simulink model "Speed_Control_Scalar"  (R2023b)
settings: Solver=ode3  StartTime=0.0  StopTime=20  FixedStep=1e-5  RelTol=1e-3
libraries: spsIGBTDiodeLib x6, spsCurrentMeasurementLib x3, spsAsynchronousMachineSIUnitsLib x1, spsDCVoltageSourceLib x1, slpidlib x1, simulink x1, spspowerguiLib x1
settings Model: Creator=G Nithish Chandra  LastModifiedBy=G Nithish Chandra

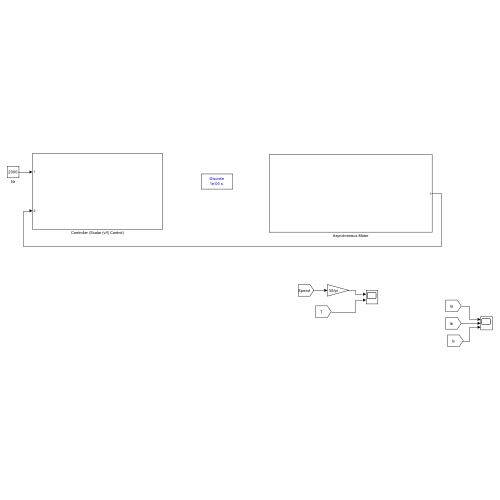
[thumbnail: Simulink's stored preview of the top-level diagram]
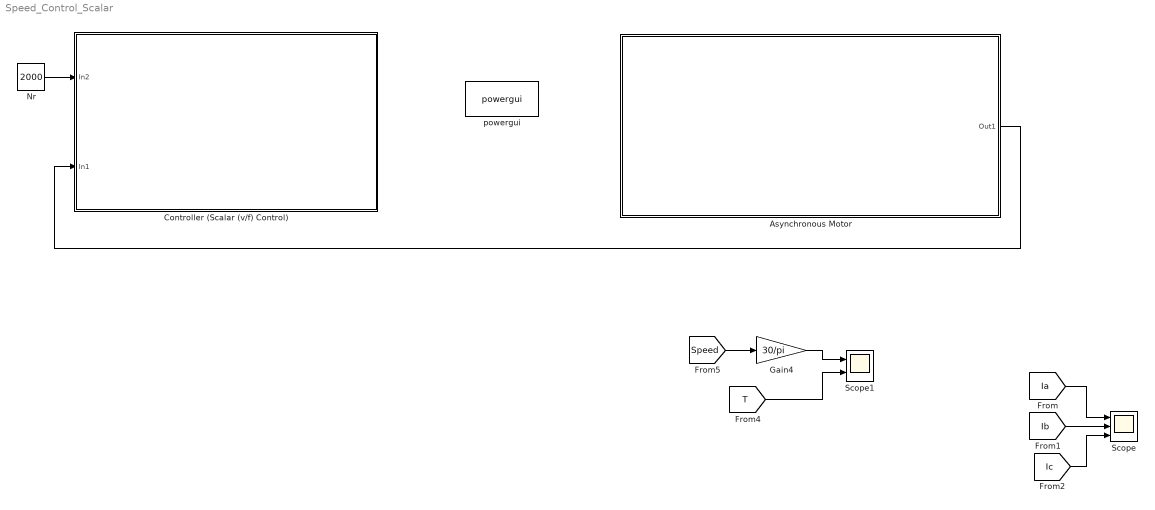
== system Speed_Control_Scalar ==
  Asynchronous Motor : Subsystem
  Controller (Scalar (v/f) Control) : Subsystem
  Gain4 : Gain  Gain=30/pi
  Nr : Constant  Value=2000
  Scope : Scope  NumInputPorts=3
  Scope1 : Scope  NumInputPorts=2
  powergui : spspowerguiLib/powergui  Priority=1  SimulationMode=Discrete  SampleTime=1e-5  frequency=60  Iterations=50  frequencyindice=50  Pbase=100e6  ErrMax=1e-4  UnitsV=kV  UnitsW=MW  buscounter=0  FunctionMessages=off  echomessages=off  EnableUseOfTLC=off  CurrentSourceSwitches=off  DisableSnubberDevices=off  DisableRonSwitches=off  DisableVfSwitches=off  DisplayEquations=off  AutomaticDiscreteSolvers=off  SolverType=Tustin/Backward Euler (TBE)  Interpol=off  ExternalGateDelay=off  methode=off  Ts=100  x0status=blocks  SPID=on  SwTol=0  HookPort=off  NonlinearTolerance=1e-4  nMaxIteration=100  ContinueOnMaxIteration=off  RestoreLinks=warning  ResistiveCurrentMeasurement=off  Frange=[0:2:500]  Ylog=off  Xlog=on  ShowGrid=off  save=off  variable=ZData  structure=0  ZoomFFT=off  StartTime=0.0  cycles=1  DisplayStyle=1  fundamental=60  FreqAxis=off  MaxFrequency=1000  frequencyindicesteady=1  RmsSteady=1  display=off
  wires:
  [Ia] -> Scope/1
  [Ic] -> Scope/3
  [Ib] -> Scope/2
  Asynchronous Motor/1(Out1) -> Controller (Scalar (v/f) Control)/2(In1)
  Nr/1 -> Controller (Scalar (v/f) Control)/1(In2)
  [Speed] -> Gain4/1
  Gain4/1 -> Scope1/1
  [T] -> Scope1/2

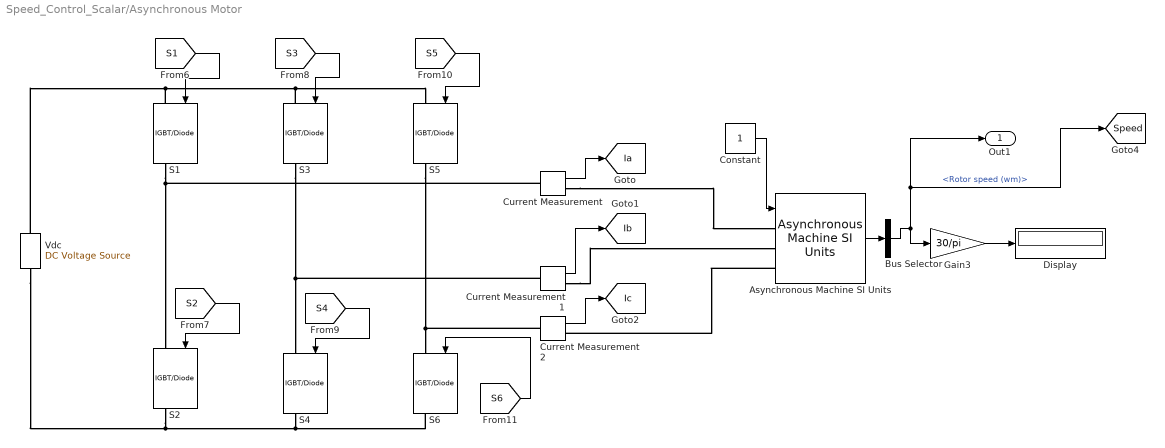
== system Speed_Control_Scalar/Asynchronous Motor ==
  Asynchronous Machine SI Units : spsAsynchronousMachineSIUnitsLib/Asynchronous Machine SI Units  RotorType=Squirrel-cage  PresetModel=No  MechanicalLoad=Torque Tm  ShowDetailedParameters=on  ReferenceFrame=Rotor  Units=SI  MeasurementBus=off  NominalParameters=[1.845e+04 400 50]  VoltageRatio=1  Stator=[0.5968 0.0003495]  Rotor=[0.6258 0.005473]  Cage1=[0.4155 0.002066]  Cage2=[0.4168 0.0003495]  Lm=0.0354  Mechanical=[0.05 0.005879 2]  PolePairs=2  InitialConditions=[0 0 0 0 0 0 0 0]  SimulateSaturation=off  Saturation=[14.03593122, 27.81365428, 53.79336849, 72.68890987, 97.98006896, 148.6815601, 215.7428561, 302.9841135, 428.7778367 ; 230, 322, 414, 460, 506, 552, 598, 644, 690]  LoadFlowParameters=1492000  TsPowergui=0  TsBlock=-1  IterativeModel=Trapezoidal non iterative  IterativeDiscreteModel=Trapezoidal non iterative  Pmec=1.492e+006
  Bus Selector : BusSelector  OutputSignals=Mechanical.Rotor speed (wm)
  Constant : Constant
  Current Measurement : spsCurrentMeasurementLib/Current Measurement  PhasorSimulation=off  OutputType=Complex  PSBequivalent=0
  Current Measurement1 : spsCurrentMeasurementLib/Current Measurement  PhasorSimulation=off  OutputType=Complex  PSBequivalent=0
  Current Measurement2 : spsCurrentMeasurementLib/Current Measurement  PhasorSimulation=off  OutputType=Complex  PSBequivalent=0
  Display : Display
  Gain3 : Gain  Gain=30/pi
  S{1..6} (6 alike) : spsIGBTDiodeLib/IGBT//Diode  Ron=1e-3  Rs=1e5  Cs=inf  Measurements=on
  Vdc : spsDCVoltageSourceLib/DC Voltage Source  Amplitude=100  Measurements=None
  Out1 : Outport
  tag scope: Ia=global, Ib=global, Ic=global, Speed=global
  wires:
  [S6] -> S6/1
  Current Measurement1/1 -> [Ib]
  Gain3/1 -> Display/1
  [S2] -> S2/1
  Constant/1 -> Asynchronous Machine SI Units/1
  [S3] -> S3/1
  Asynchronous Machine SI Units/1 -> Bus Selector/1
  Bus Selector/1 -> [Speed], Out1/1, Gain3/1  "<Rotor speed (wm)>"
  [S4] -> S4/1
  [S5] -> S5/1
  Current Measurement/1 -> [Ia]
  [S1] -> S1/1
  Current Measurement2/1 -> [Ic]
  connections:
  S2/RConn1 -- Vdc/LConn1 -- S4/RConn1 -- S6/RConn1
  Current Measurement1/RConn1 -- Asynchronous Machine SI Units/LConn2
  S5/RConn1 -- Current Measurement2/LConn1 -- S6/LConn1
  S3/RConn1 -- Current Measurement1/LConn1 -- S4/LConn1
  Current Measurement/RConn1 -- Asynchronous Machine SI Units/LConn1
  S1/RConn1 -- S2/LConn1 -- Current Measurement/LConn1
  S1/LConn1 -- S3/LConn1 -- S5/LConn1 -- Vdc/RConn1
  Asynchronous Machine SI Units/LConn3 -- Current Measurement2/RConn1

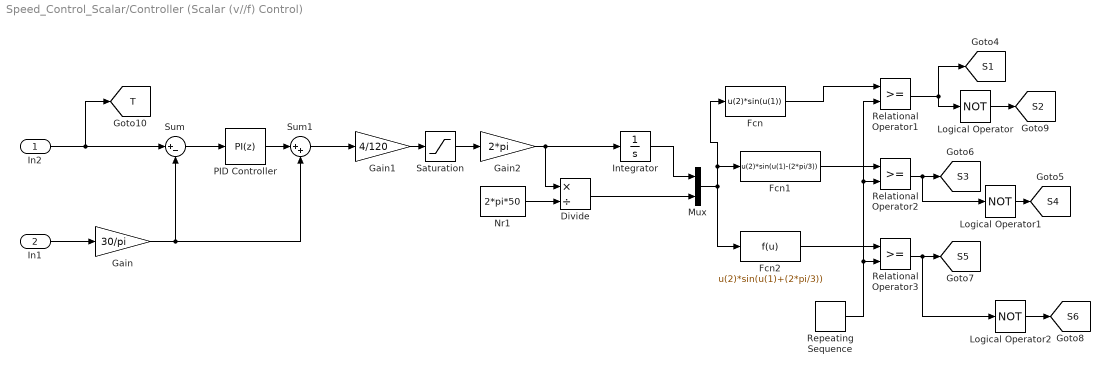
== system Speed_Control_Scalar/Controller (Scalar (v//f) Control) ==
  In2 : Inport
  In1 : Inport  Port=2
  Divide : Product  Inputs=*/
  Fcn : Fcn  Expr=u(2)*sin(u(1))
  Fcn1 : Fcn  Expr=u(2)*sin(u(1)-(2*pi/3))
  Fcn2 : Fcn  Expr=u(2)*sin(u(1)+(2*pi/3))
  Gain : Gain  Gain=30/pi
  Gain1 : Gain  Gain=4/120
  Gain2 : Gain  Gain=2*pi
  Integrator : Integrator
  Logical Operator : Logic  Operator=NOT  AllPortsSameDT=off  OutDataTypeStr=boolean
  Logical Operator1 : Logic  Operator=NOT  AllPortsSameDT=off  OutDataTypeStr=boolean
  Logical Operator2 : Logic  Operator=NOT  AllPortsSameDT=off  OutDataTypeStr=boolean
  Mux : Mux  Inputs=2
  Nr1 : Constant  Value=2*pi*50
  PID Controller : slpidlib/PID Controller  Controller=PI  Form=Parallel  TimeDomain=Discrete-time  UseExternalTs=off  SampleTime=1e-5  IntegratorMethod=Forward Euler  FilterMethod=Forward Euler  ControllerParametersSource=internal  P=1  I=1  UseKiTs=off  D=0  N=100  UseFilter=on  TunerSelectOption=Transfer Function Based (PID Tuner App)  InitialConditionSource=internal  InitialConditionForIntegrator=0  InitialConditionForFilter=0  DifferentiatorICPrevScaledInput=0  ExternalReset=none  TrackingMode=off  Kt=1  LimitOutput=off  SatLimitsSource=internal  UpperSaturationLimit=inf  LowerSaturationLimit=-inf  LinearizeAsGain=on  AntiWindupMode=none  Kb=1  LimitIntegrator=off  UpperIntegratorSaturationLimit=inf  LowerIntegratorSaturationLimit=-inf  POutMin=[]  POutMax=[]  IOutMin=[]  IOutMax=[]  DOutMin=[]  DOutMax=[]  NOutMin=[]  NOutMax=[]  SumOutMin=[]  SumOutMax=[]  SaturationOutMin=[]  SaturationOutMax=[]  PParamMin=[]  PParamMax=[]  IParamMin=[]  IParamMax=[]  DParamMin=[]  DParamMax=[]  NParamMin=[]  NParamMax=[]  KbParamMin=[]  KbParamMax=[]  KtParamMin=[]  KtParamMax=[]  KbOutMin=[]  KbOutMax=[]  KtOutMin=[]  KtOutMax=[]  IntegratorOutMin=[]  IntegratorOutMax=[]  FilterOutMin=[]  FilterOutMax=[]  SumI1OutMin=[]  SumI1OutMax=[]  SumI2OutMin=[]  SumI2OutMax=[]  SumI3OutMin=[]  SumI3OutMax=[]  SumI4OutMin=[]  SumI4OutMax=[]  SumDOutMin=[]  SumDOutMax=[]  DifferentiatorOutMin=[]  DifferentiatorOutMax=[]  FilterDiffOutCoefMin=[]  FilterDiffOutCoefMax=[]  ReciprocalOutMin=[]  ReciprocalOutMax=[]  SumDenOutMin=[]  SumDenOutMax=[]  SumNumOutMin=[]  SumNumOutMax=[]  DivideOutMin=[]  DivideOutMax=[]  UdiffTsProdOutMin=[]  UdiffTsProdOutMax=[]  NTsProdOutMin=[]  NTsProdOutMax=[]  UintegralTsProdOutMin=[]  UintegralTsProdOutMax=[]  UngainTsProdOutMin=[]  UngainTsProdOutMax=[]  ClampingZeroOutDataTypeStr=Inherit: Inherit via back propagation  ClampingZeroOutMin=[]  ClampingZeroOutMax=[]  FilterDenConstantOutDataTypeStr=Inherit: Inherit via back propagation  FilterDenConstantOutMin=[]  FilterDenConstantOutMax=[]  PCopyOutDataTypeStr=Inherit: Inherit via back propagation  PCopyOutMin=[]  PCopyOutMax=[]  NCopyOutDataTypeStr=Inherit: Inherit via back propagation  NCopyOutMin=[]  NCopyOutMax=[]  IntegratorContinuousStateAttributes=''  IntegratorStateMustResolveToSignalObject=off  IntegratorRTWStateStorageClass=Auto  FilterContinuousStateAttributes=''  FilterStateMustResolveToSignalObject=off  FilterRTWStateStorageClass=Auto  ParallelPVariant=InternalParameters  IdealPVariant=Disabled  IVariant=InternalParameters  DVariant=Disabled  IntegratorVariant=Discrete  SatVariant=Disabled  AWVariant=Passthrough  PCopyVariant=Disabled  TRVariant=Disabled  FdbkBlocksVariant=Forward  IdealPFdbkVariant=Disabled  SatFdbkVariant=Disabled  DerivativeFilterVariant=Disabled  NVariant=Disabled  NCopyVariant=Disabled_SignalSpec  FilterICVariant=Disabled  IntegratorICVariant=InternalICs  ExternalResetVariant=Disabled  TRSumVariant=Passthrough  SumFdbkVariant=Disabled  SumVariant=Sum_PI  TsampFilterVariant=InternalTs  TsampNgainVariant=Passthrough  TsampIntegralVariant=Disabled_SignalSpec  ExternalSaturationOutDataTypeStr=Inherit: Same as second input
  Relational Operator1 : RelationalOperator  OutDataTypeStr=boolean  RndMeth=Simplest  InputSameDT=off
  Relational Operator2 : RelationalOperator  OutDataTypeStr=boolean  RndMeth=Simplest  InputSameDT=off
  Relational Operator3 : RelationalOperator  OutDataTypeStr=boolean  RndMeth=Simplest  InputSameDT=off
  Repeating Sequence : simulink/Sources/Repeating Sequence  rep_seq_t=[0 1 2]*(1/5000)  rep_seq_y=[-1 1 -1 ]
  Saturation : Saturate  UpperLimit=50  LowerLimit=0
  Sum : Sum  Inputs=|+-
  Sum1 : Sum  Inputs=|++
  tag scope: S1=global, S2=global, S3=global, S4=global, S5=global, S6=global, T=global
  wires:
  In2/1 -> [T], Sum/1
  Gain1/1 -> Saturation/1
  Sum1/1 -> Gain1/1
  In1/1 -> Gain/1
  Sum/1 -> PID Controller/1
  Gain/1 -> Sum1/2, Sum/2
  Logical Operator2/1 -> [S6]
  PID Controller/1 -> Sum1/1
  Gain2/1 -> Integrator/1, Divide/1
  Saturation/1 -> Gain2/1
  Fcn2/1 -> Relational Operator3/1
  Mux/1 -> Fcn1/1, Fcn/1, Fcn2/1
  Relational Operator1/1 -> [S1], Logical Operator/1
  Fcn/1 -> Relational Operator1/1
  Integrator/1 -> Mux/1
  Divide/1 -> Mux/2
  Nr1/1 -> Divide/2
  Relational Operator3/1 -> Logical Operator2/1, [S5]
  Relational Operator2/1 -> Logical Operator1/1, [S3]
  Repeating Sequence/1 -> Relational Operator3/2, Relational Operator2/2, Relational Operator1/2
  Logical Operator1/1 -> [S4]
  Fcn1/1 -> Relational Operator2/1
  Logical Operator/1 -> [S2]
